simulink model "LAB 8 pcm"  (R2014b)
settings: Solver=ode45  StartTime=0.0  StopTime=5  RelTol=1e-3
libraries: commutil2 x2, dspquant2 x2, dsparch4 x1, dspsigops x1
settings Model: Creator=admin  LastModifiedBy=admin

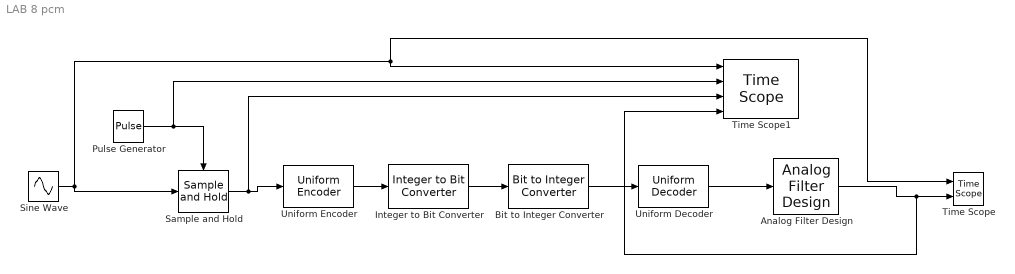
== system LAB 8 pcm ==
  Analog Filter Design : dsparch4/Analog Filter Design  method=Butterworth  filttype=Lowpass  N=8  Wlo=2*pi  Whi=80  Rp=2  Rs=40
  Bit to Integer Converter : commutil2/Bit to Integer Converter  nbits=3  bitOrder=MSB first  signedOutputValues=Signed  outDtype=Inherit via internal rule  outDtypeSigned=Inherit via internal rule
  Integer to Bit Converter : commutil2/Integer to Bit Converter  nbits=3  signedInputValues=Signed  bitOrder=MSB first  outDtype=Inherit via internal rule
  Pulse Generator : DiscretePulseGenerator  PulseType=Time based  Amplitude=5  Period=1/20  PulseWidth=50
  Sample and Hold : dspsigops/Sample and Hold  trig=Rising edge  initCond=0  latchinput=off
  Sine Wave : Sin  Amplitude=5  Frequency=2*pi  SampleTime=0.01
  Time Scope : TimeScope  DefaultConfigurationName=spbscopes.TimeScopeBlockCfg  NumInputPorts=2
  Time Scope1 : TimeScope  DefaultConfigurationName=spbscopes.TimeScopeBlockCfg  NumInputPorts=4
  Uniform Decoder : dspquant2/Uniform Decoder  peak=1  bits=3  overflowMode=Saturate  otype=Double
  Uniform Encoder : dspquant2/Uniform Encoder  peak=5  bits=3  otype=Signed integer
  wires:
  Pulse Generator/1 -> Time Scope1/2, Sample and Hold/Trigger
  Sine Wave/1 -> Time Scope/1, Time Scope1/1, Sample and Hold/1
  Sample and Hold/1 -> Time Scope1/3, Uniform Encoder/1
  Integer to Bit Converter/1 -> Bit to Integer Converter/1
  Bit to Integer Converter/1 -> Uniform Decoder/1
  Uniform Decoder/1 -> Analog Filter Design/1
  Analog Filter Design/1 -> Time Scope1/4, Time Scope/2
  Uniform Encoder/1 -> Integer to Bit Converter/1
